simulink model "design_pid_controller"  (R2024a)
settings: Solver=VariableStepAuto  StartTime=0.0  StopTime=10.0  RelTol=1e-3
values from neighbouring files (symbols this model uses):
  B = 1.4411e-4    (= 0.00014411)    [estimated_parameters.m]    (also in inital_parameters.m = 0.00015)
  J = 2.657e-5    (= 2.657e-05)    [estimated_parameters.m]    (also in inital_parameters.m = 9.76e-05)
  Kb = 0.0062    [estimated_parameters.m]    (also in inital_parameters.m = 0.00768)
  Km = 0.0561    [estimated_parameters.m]    (also in inital_parameters.m = 0.00768)
  L = 0.18e-3    (= 0.00018)    [estimated_parameters.m]    (also in inital_parameters.m)
  R = 4.9476    [estimated_parameters.m]    (also in inital_parameters.m = 10)
libraries: slpidlib x1
settings Model: Creator=mashr  LastModifiedBy=mashr

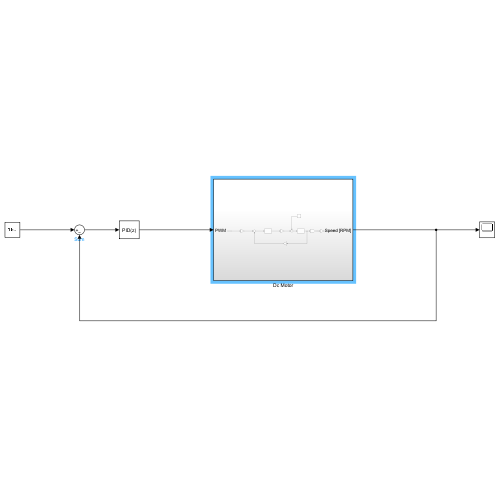
[thumbnail: Simulink's stored preview of the top-level diagram]
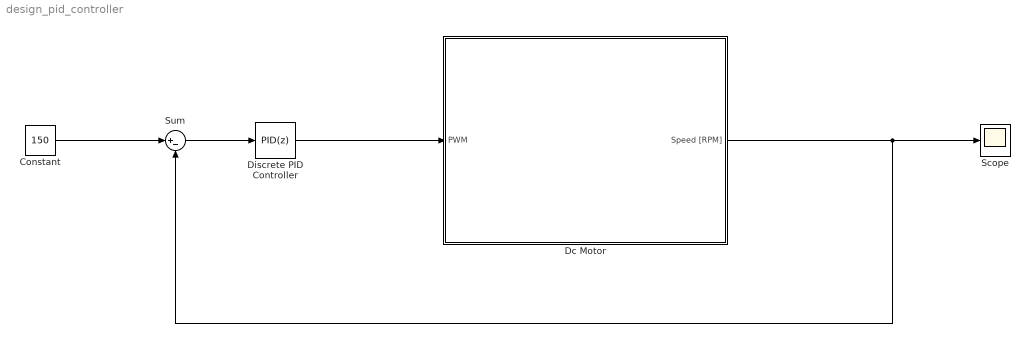
== system design_pid_controller ==
  Constant : Constant  Value=150  SampleTime=0.001
  Dc Motor : Subsystem
  Discrete PID Controller : slpidlib/PID Controller  Controller=PID  Form=Parallel  TimeDomain=Discrete-time  UseExternalTs=off  SampleTime=-1  IntegratorMethod=Forward Euler  FilterMethod=Forward Euler  ControllerParametersSource=internal  P=0.6878985173518  I=5.48570531959692  UseKiTs=off  D=0  UseExternalDerivativeSource=off  N=100  UseFilter=on  TunerSelectOption=Transfer Function Based (PID Tuner App)  InitialConditionSource=internal  InitialConditionForIntegrator=0  InitialConditionForFilter=0  DifferentiatorICPrevScaledInput=0  ExternalReset=none  TrackingMode=off  Kt=1  LimitOutput=off  SatLimitsSource=internal  UpperSaturationLimit=inf  LowerSaturationLimit=-inf  LinearizeAsGain=off  AntiWindupMode=none  Kb=1  LimitIntegrator=off  UpperIntegratorSaturationLimit=inf  LowerIntegratorSaturationLimit=-inf  POutMin=[]  POutMax=[]  IOutMin=[]  IOutMax=[]  DOutMin=[]  DOutMax=[]  NOutMin=[]  NOutMax=[]  SumOutMin=[]  SumOutMax=[]  SaturationOutMin=[]  SaturationOutMax=[]  PParamMin=[]  PParamMax=[]  IParamMin=[]  IParamMax=[]  DParamMin=[]  DParamMax=[]  NParamMin=[]  NParamMax=[]  KbParamMin=[]  KbParamMax=[]  KtParamMin=[]  KtParamMax=[]  KbOutMin=[]  KbOutMax=[]  KtOutMin=[]  KtOutMax=[]  IntegratorOutMin=[]  IntegratorOutMax=[]  FilterOutMin=[]  FilterOutMax=[]  SumI1OutMin=[]  SumI1OutMax=[]  SumI2OutMin=[]  SumI2OutMax=[]  SumI3OutMin=[]  SumI3OutMax=[]  SumI4OutMin=[]  SumI4OutMax=[]  SumDOutMin=[]  SumDOutMax=[]  DifferentiatorOutMin=[]  DifferentiatorOutMax=[]  FilterDiffOutCoefMin=[]  FilterDiffOutCoefMax=[]  ReciprocalOutMin=[]  ReciprocalOutMax=[]  SumDenOutMin=[]  SumDenOutMax=[]  SumNumOutMin=[]  SumNumOutMax=[]  DivideOutMin=[]  DivideOutMax=[]  UdiffTsProdOutMin=[]  UdiffTsProdOutMax=[]  NTsProdOutMin=[]  NTsProdOutMax=[]  UintegralTsProdOutMin=[]  UintegralTsProdOutMax=[]  UngainTsProdOutMin=[]  UngainTsProdOutMax=[]  ClampingZeroOutDataTypeStr=Inherit: Inherit via back propagation  ClampingZeroOutMin=[]  ClampingZeroOutMax=[]  FilterDenConstantOutDataTypeStr=Inherit: Inherit via back propagation  FilterDenConstantOutMin=[]  FilterDenConstantOutMax=[]  PCopyOutDataTypeStr=Inherit: Inherit via back propagation  PCopyOutMin=[]  PCopyOutMax=[]  NCopyOutDataTypeStr=Inherit: Inherit via back propagation  NCopyOutMin=[]  NCopyOutMax=[]  IntegratorContinuousStateAttributes=''  IntegratorStateMustResolveToSignalObject=off  IntegratorRTWStateStorageClass=Auto  FilterContinuousStateAttributes=''  FilterStateMustResolveToSignalObject=off  FilterRTWStateStorageClass=Auto  ParallelPVariant=InternalParameters  IdealPVariant=Disabled  IVariant=InternalParameters  DVariant=InternalParameters  IntegratorVariant=Discrete  SatVariant=Disabled  AWVariant=Passthrough  PCopyVariant=Disabled  TRVariant=Disabled  FdbkBlocksVariant=Forward  IdealPFdbkVariant=Disabled  SatFdbkVariant=Disabled  DerivativeFilterVariant=ForwardEulerFilter  NVariant=InternalParameters  NCopyVariant=Disabled  FilterICVariant=InternalICsFilter  IntegratorICVariant=InternalICs  ExternalResetVariant=Disabled  TRSumVariant=Passthrough  SumFdbkVariant=Disabled  SumVariant=Sum_PID  TsampFilterVariant=InternalTs  TsampNgainVariant=Passthrough  TsampIntegralVariant=Disabled_SignalSpec  ExternalSaturationOutDataTypeStr=Inherit: Same as second input  DerivativeSourceVariant=ErrorSignal
      settings: LibrarySourceBlock=simulink/Discrete/Discrete PID Controller
  Scope : Scope
  Sum : Sum  Inputs=|+-
  wires:
  Discrete PID Controller/1 -> Dc Motor/1(PWM)
  Sum/1 -> Discrete PID Controller/1
  Dc Motor/1(Speed [RPM]) -> Scope/1, Sum/2
  Constant/1 -> Sum/1

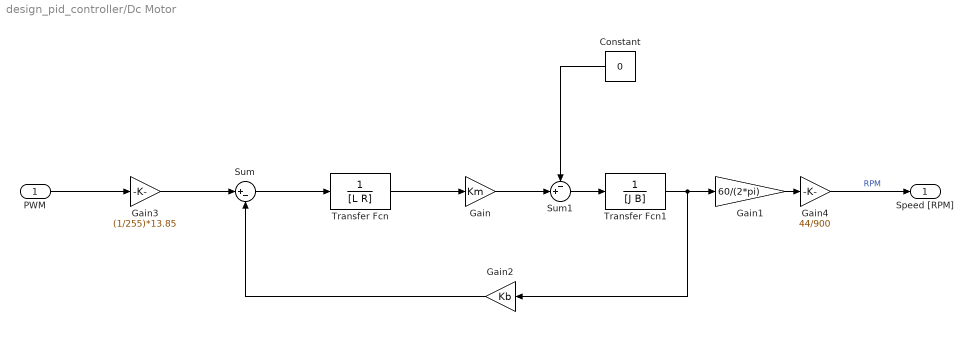
== system design_pid_controller/Dc Motor ==
  PWM : Inport
  Constant : Constant  Value=0  SampleTime=0.01
  Gain : Gain  Gain=Km
  Gain1 : Gain  Gain=60/(2*pi)  OutDataTypeStr=double
  Gain2 : Gain  Gain=Kb
  Gain3 : Gain  Gain=(1/255)*13.85  OutDataTypeStr=double
  Gain4 : Gain  Gain=44/900  OutDataTypeStr=double
  Sum : Sum  Inputs=|+-
  Sum1 : Sum  Inputs=-+|
  Transfer Fcn : TransferFcn  Denominator=[L R]
  Transfer Fcn1 : TransferFcn  Denominator=[J B]
  Speed [RPM] : Outport
  wires:
  Transfer Fcn/1 -> Gain/1
  Sum1/1 -> Transfer Fcn1/1
  Gain/1 -> Sum1/2
  Transfer Fcn1/1 -> Gain1/1, Gain2/1
  Gain3/1 -> Sum/1
  Constant/1 -> Sum1/1
  Gain1/1 -> Gain4/1
  Sum/1 -> Transfer Fcn/1
  Gain4/1 -> Speed [RPM]/1  "RPM"
  Gain2/1 -> Sum/2
  PWM/1 -> Gain3/1
